simulink model "es2_sim_rimolo"  (R2023a)
settings: Solver=VariableStepAuto  StartTime=0.0  StopTime=10.0  RelTol=1e-3
undefined symbols (not defined in the file or in its folder): Alin, Blin, Clin, ueq, x0, xeq1
settings Model: Creator=Admin  LastModifiedBy=Admin

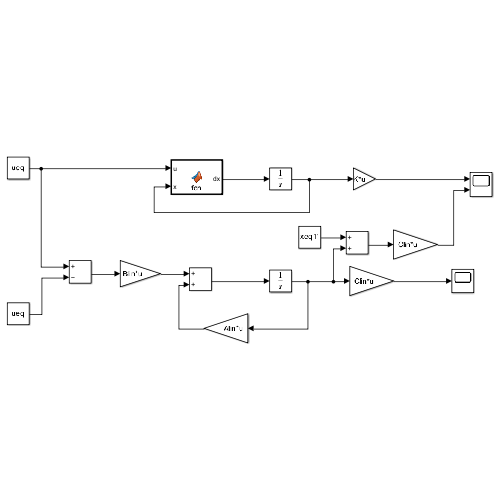
[thumbnail: Simulink's stored preview of the top-level diagram]
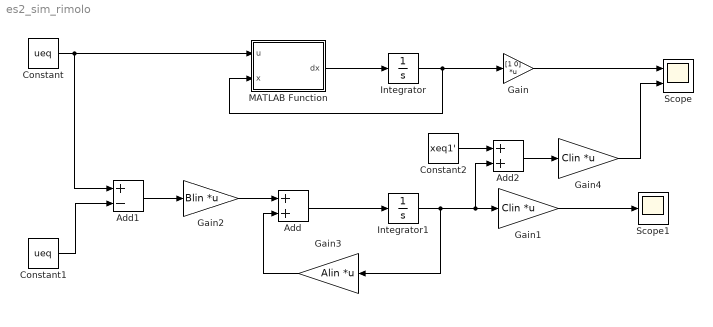
== system es2_sim_rimolo ==
  Add : Sum
  Add1 : Sum  Inputs=+-
  Add2 : Sum
  Constant : Constant  Value=ueq
  Constant1 : Constant  Value=ueq
  Constant2 : Constant  Value=xeq1'
  Gain : Gain  Gain=[1 0]  Multiplication=Matrix(K*u)
  Gain1 : Gain  Gain=Clin  Multiplication=Matrix(K*u)
  Gain2 : Gain  Gain=Blin  Multiplication=Matrix(K*u)
  Gain3 : Gain  Gain=Alin  Multiplication=Matrix(K*u)
  Gain4 : Gain  Gain=Clin  Multiplication=Matrix(K*u)
  Integrator : Integrator  InitialCondition=x0
  Integrator1 : Integrator  InitialCondition=x0-xeq1'
  MATLAB Function : MATLAB Function  TreatAsAtomicUnit=on
  Scope : Scope  NumInputPorts=2
  Scope1 : Scope
  wires:
  MATLAB Function/1(dx) -> Integrator/1
  Integrator/1 -> Gain/1, MATLAB Function/2(x)
  Constant/1 -> Add1/1, MATLAB Function/1(u)
  Gain/1 -> Scope/1
  Add/1 -> Integrator1/1
  Integrator1/1 -> Gain3/1, Add2/2, Gain1/1
  Gain2/1 -> Add/1
  Gain3/1 -> Add/2
  Add1/1 -> Gain2/1
  Constant1/1 -> Add1/2
  Gain1/1 -> Scope1/1
  Constant2/1 -> Add2/1
  Add2/1 -> Gain4/1
  Gain4/1 -> Scope/2

== matlab function es2_sim_rimolo/MATLAB Function ==
  data: u input; dx output; x input
function dx = fcn(u,x)

x1=x(1);
x2=x(2);
dx=[x1*(0.01*x1-1)+(x1*x2)/50;0.001*x1*x2/1000-0.1*x2+u];
